simulink model "SS_Extended_Est"  (R2021a)
settings: Solver=ode45  StartTime=0.0  StopTime=1  RelTol=1e-3
undefined symbols (not defined in the file): drv, est_par, gbox, mot, rads2rpm, sens, ss_est
settings Model: Creator=gioel  LastModifiedBy=gioel
settings DataIOCC: ReturnWorkspaceOutputs=off

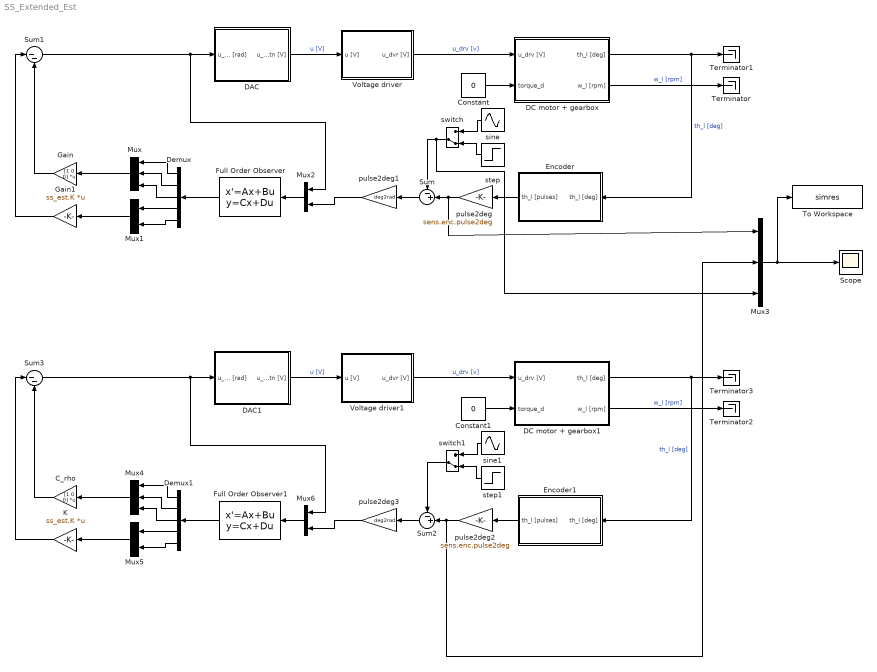
== system SS_Extended_Est ==
  C_rho : Gain  Gain=[1 0 0]  Multiplication=Matrix(K*u)
  Constant : Constant  Value=0
  Constant1 : Constant  Value=0
  DAC : Subsystem
  DAC1 : Subsystem
  DC motor + gearbox : Subsystem
  DC motor + gearbox1 : Subsystem
  Demux : Demux  Outputs=5
  Demux1 : Demux  Outputs=5
  Encoder : Subsystem
  Encoder1 : Subsystem
  Full Order Observer : StateSpace  A=ss_est.Ae_3 - ss_est.Le_3*ss_est.Ce  B=[ss_est.Be ss_est.Le_3]  C=eye(5)  D=[0 0; 0 0;0 0;0 0;0 0]  InitialCondition=0
  Full Order Observer1 : StateSpace  A=ss_est.Ae_3 - ss_est.Le_3*ss_est.Ce  B=[ss_est.Be ss_est.Le_3]  C=eye(5)  D=[0 0; 0 0;0 0;0 0;0 0]  InitialCondition=0
  Gain : Gain  Gain=[1 0 0]  Multiplication=Matrix(K*u)
  Gain1 : Gain  Gain=ss_est.K  Multiplication=Matrix(K*u)
  K : Gain  Gain=ss_est.K  Multiplication=Matrix(K*u)
  Mux : Mux  Inputs=3
  Mux{1..2,5..6} (4 alike) : Mux  Inputs=2
  Mux3 : Mux  Inputs=3
  Mux4 : Mux  Inputs=3
  Scope : Scope
  Sum : Sum  Inputs=-+|
  Sum1 : Sum  Inputs=|--
  Sum2 : Sum  Inputs=-+|
  Sum3 : Sum  Inputs=|--
  Terminator{,1..3} (4 alike) : Terminator
  To Workspace : ToWorkspace  VariableName=simres  SaveFormat=Structure With Time  SampleTime=-1
  Voltage driver : Subsystem
  Voltage driver1 : Subsystem
  pulse2deg : Gain  Gain=sens.enc.pulse2deg
  pulse2deg1 : Gain  Gain=deg2rad
  pulse2deg2 : Gain  Gain=sens.enc.pulse2deg
  pulse2deg3 : Gain  Gain=deg2rad
  sine : Sin  Amplitude=40  Frequency=2*pi/0.1  SampleTime=0
  sine1 : Sin  Amplitude=40  Frequency=2*pi/0.1  SampleTime=0
  step : Step  Time=0  After=40  SampleTime=0
  step1 : Step  Time=0  After=40  SampleTime=0
  switch : ManualSwitch  CurrentSetting=0
  switch1 : ManualSwitch  CurrentSetting=0
  wires:
  DC motor + gearbox/2(w_l [rpm]) -> Terminator/1  "w_l [rpm]"
  Voltage driver/1(u_dvr [V]) -> DC motor + gearbox/1(u_drv [V])  "u_drv [v]"
  Constant/1 -> DC motor + gearbox/2(torque_d)
  Encoder/1(th_l [pulses]) -> pulse2deg/1
  DAC/1(u_cntn [V]) -> Voltage driver/1(u [V])  "u [V]"
  Sum1/1 -> Mux2/1, DAC/1(u_dscr [rad])
  DC motor + gearbox/1(th_l [deg]) -> Terminator1/1, Encoder/1(th_l [deg])  "th_l [deg]"
  pulse2deg/1 -> Mux3/1, Sum/2
  Full Order Observer/1 -> Demux/1
  Demux/2 -> Mux/2
  Demux/1 -> Mux/1
  Demux/3 -> Mux/3
  Demux/4 -> Mux1/1
  Demux/5 -> Mux1/2
  Gain/1 -> Sum1/2
  Mux/1 -> Gain/1
  Sum/1 -> pulse2deg1/1
  pulse2deg1/1 -> Mux2/2
  Mux1/1 -> Gain1/1
  Gain1/1 -> Sum1/1
  Mux2/1 -> Full Order Observer/1
  sine/1 -> switch/1
  step/1 -> switch/2
  switch/1 -> Mux3/3, Sum/1
  switch1/1 -> Sum2/1
  step1/1 -> switch1/2
  sine1/1 -> switch1/1
  Mux6/1 -> Full Order Observer1/1
  K/1 -> Sum3/1
  Mux5/1 -> K/1
  pulse2deg3/1 -> Mux6/2
  Sum2/1 -> pulse2deg3/1
  Mux4/1 -> C_rho/1
  C_rho/1 -> Sum3/2
  Demux1/5 -> Mux5/2
  Demux1/4 -> Mux5/1
  Demux1/3 -> Mux4/3
  Demux1/1 -> Mux4/1
  Demux1/2 -> Mux4/2
  Full Order Observer1/1 -> Demux1/1
  pulse2deg2/1 -> Sum2/2, Mux3/2
  DC motor + gearbox1/1(th_l [deg]) -> Encoder1/1(th_l [deg]), Terminator3/1  "th_l [deg]"
  Sum3/1 -> DAC1/1(u_dscr [rad]), Mux6/1
  DAC1/1(u_cntn [V]) -> Voltage driver1/1(u [V])  "u [V]"
  Encoder1/1(th_l [pulses]) -> pulse2deg2/1
  Constant1/1 -> DC motor + gearbox1/2(torque_d)
  Voltage driver1/1(u_dvr [V]) -> DC motor + gearbox1/1(u_drv [V])  "u_drv [v]"
  DC motor + gearbox1/2(w_l [rpm]) -> Terminator2/1  "w_l [rpm]"
  Mux3/1 -> Scope/1, To Workspace/1

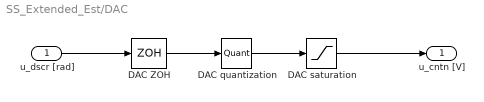
== system SS_Extended_Est/DAC ==
  u_dscr [rad] : Inport
  DAC ZOH : ZeroOrderHold  SampleTime=sens.enc.T_s
  DAC quantization : Quantizer  QuantizationInterval=daq.dac.q
  DAC saturation : Saturate  UpperLimit=10  LowerLimit=-10
  u_cntn [V] : Outport
  wires:
  DAC quantization/1 -> DAC saturation/1
  DAC ZOH/1 -> DAC quantization/1
  DAC saturation/1 -> u_cntn [V]/1
  u_dscr [rad]/1 -> DAC ZOH/1

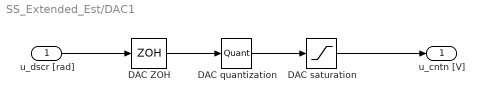
== system SS_Extended_Est/DAC1 ==
  u_dscr [rad] : Inport
  DAC ZOH : ZeroOrderHold  SampleTime=sens.enc.T_s
  DAC quantization : Quantizer  QuantizationInterval=daq.dac.q
  DAC saturation : Saturate  UpperLimit=10  LowerLimit=-10
  u_cntn [V] : Outport
  wires:
  u_dscr [rad]/1 -> DAC ZOH/1
  DAC saturation/1 -> u_cntn [V]/1
  DAC ZOH/1 -> DAC quantization/1
  DAC quantization/1 -> DAC saturation/1

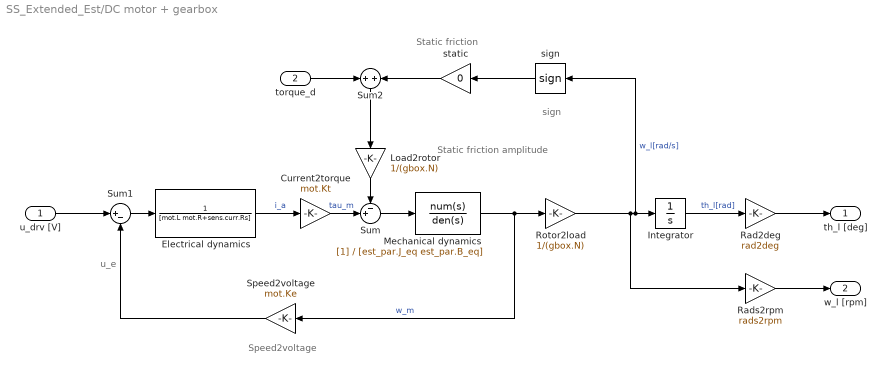
== system SS_Extended_Est/DC motor + gearbox ==
  note: u_e
  note: Speed2voltage
  note: Static friction
  note: sign
  note: Static friction
      |  amplitude
  u_drv [V] : Inport
  torque_d : Inport  Port=2
  Current2torque : Gain  Gain=mot.Kt
  Electrical dynamics : TransferFcn  Denominator=[mot.L mot.R+sens.curr.Rs]
  Integrator : Integrator
  Load2rotor : Gain  Gain=1/(gbox.N)
  Mechanical dynamics : TransferFcn  Denominator=[est_par.J_eq est_par.B_eq]
  Rad2deg : Gain  Gain=rad2deg
  Rads2rpm : Gain  Gain=rads2rpm
  Rotor2load : Gain  Gain=1/(gbox.N)
  Speed2voltage : Gain  Gain=mot.Ke
  Sum : Sum  Inputs=-+|
  Sum1 : Sum  Inputs=|+-
  Sum2 : Sum  Inputs=+|+
  sign : Signum  ZeroCross=off
  static : Gain  Gain=0
  th_l [deg] : Outport
  w_l [rpm] : Outport  Port=2
  wires:
  u_drv [V]/1 -> Sum1/1
  Rads2rpm/1 -> w_l [rpm]/1
  Electrical dynamics/1 -> Current2torque/1  "i_a"
  Current2torque/1 -> Sum/2  "tau_m"
  Rad2deg/1 -> th_l [deg]/1
  sign/1 -> static/1
  Sum1/1 -> Electrical dynamics/1
  Integrator/1 -> Rad2deg/1  "th_l[rad]"
  Sum/1 -> Mechanical dynamics/1
  Load2rotor/1 -> Sum/1
  Speed2voltage/1 -> Sum1/2
  Rotor2load/1 -> sign/1, Integrator/1, Rads2rpm/1  "w_l[rad/s]"
  Mechanical dynamics/1 -> Speed2voltage/1, Rotor2load/1  "w_m"
  Sum2/1 -> Load2rotor/1
  torque_d/1 -> Sum2/1
  static/1 -> Sum2/2

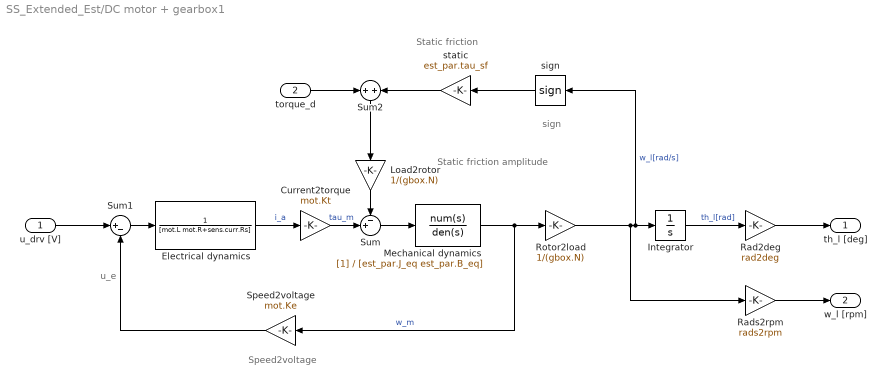
== system SS_Extended_Est/DC motor + gearbox1 ==
  note: Static friction
      |  amplitude
  note: sign
  note: Static friction
  note: Speed2voltage
  note: u_e
  u_drv [V] : Inport
  torque_d : Inport  Port=2
  Current2torque : Gain  Gain=mot.Kt
  Electrical dynamics : TransferFcn  Denominator=[mot.L mot.R+sens.curr.Rs]
  Integrator : Integrator
  Load2rotor : Gain  Gain=1/(gbox.N)
  Mechanical dynamics : TransferFcn  Denominator=[est_par.J_eq est_par.B_eq]
  Rad2deg : Gain  Gain=rad2deg
  Rads2rpm : Gain  Gain=rads2rpm
  Rotor2load : Gain  Gain=1/(gbox.N)
  Speed2voltage : Gain  Gain=mot.Ke
  Sum : Sum  Inputs=-+|
  Sum1 : Sum  Inputs=|+-
  Sum2 : Sum  Inputs=+|+
  sign : Signum  ZeroCross=off
  static : Gain  Gain=est_par.tau_sf
  th_l [deg] : Outport
  w_l [rpm] : Outport  Port=2
  wires:
  static/1 -> Sum2/2
  torque_d/1 -> Sum2/1
  Sum2/1 -> Load2rotor/1
  Mechanical dynamics/1 -> Rotor2load/1, Speed2voltage/1  "w_m"
  Rotor2load/1 -> Rads2rpm/1, Integrator/1, sign/1  "w_l[rad/s]"
  Speed2voltage/1 -> Sum1/2
  Load2rotor/1 -> Sum/1
  Sum/1 -> Mechanical dynamics/1
  Integrator/1 -> Rad2deg/1  "th_l[rad]"
  Sum1/1 -> Electrical dynamics/1
  sign/1 -> static/1
  Rad2deg/1 -> th_l [deg]/1
  Current2torque/1 -> Sum/2  "tau_m"
  Electrical dynamics/1 -> Current2torque/1  "i_a"
  Rads2rpm/1 -> w_l [rpm]/1
  u_drv [V]/1 -> Sum1/1

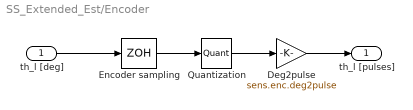
== system SS_Extended_Est/Encoder ==
  th_l [deg] : Inport
  Deg2pulse : Gain  Gain=sens.enc.deg2pulse
  Encoder sampling : ZeroOrderHold  SampleTime=0.001
  Quantization : Quantizer  QuantizationInterval=sens.enc.q
  th_l [pulses] : Outport
  wires:
  Encoder sampling/1 -> Quantization/1
  Quantization/1 -> Deg2pulse/1
  th_l [deg]/1 -> Encoder sampling/1
  Deg2pulse/1 -> th_l [pulses]/1

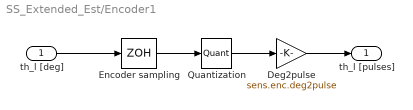
== system SS_Extended_Est/Encoder1 ==
  th_l [deg] : Inport
  Deg2pulse : Gain  Gain=sens.enc.deg2pulse
  Encoder sampling : ZeroOrderHold  SampleTime=0.001
  Quantization : Quantizer  QuantizationInterval=sens.enc.q
  th_l [pulses] : Outport
  wires:
  Deg2pulse/1 -> th_l [pulses]/1
  th_l [deg]/1 -> Encoder sampling/1
  Quantization/1 -> Deg2pulse/1
  Encoder sampling/1 -> Quantization/1

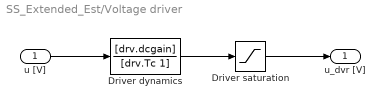
== system SS_Extended_Est/Voltage driver ==
  u [V] : Inport
  Driver dynamics : TransferFcn  Numerator=[drv.dcgain]  Denominator=[drv.Tc 1]
  Driver saturation : Saturate  UpperLimit=12  LowerLimit=-12
  u_dvr [V] : Outport
  wires:
  Driver saturation/1 -> u_dvr [V]/1
  Driver dynamics/1 -> Driver saturation/1
  u [V]/1 -> Driver dynamics/1

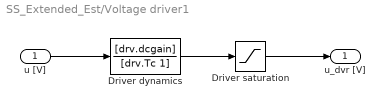
== system SS_Extended_Est/Voltage driver1 ==
  u [V] : Inport
  Driver dynamics : TransferFcn  Numerator=[drv.dcgain]  Denominator=[drv.Tc 1]
  Driver saturation : Saturate  UpperLimit=12  LowerLimit=-12
  u_dvr [V] : Outport
  wires:
  u [V]/1 -> Driver dynamics/1
  Driver dynamics/1 -> Driver saturation/1
  Driver saturation/1 -> u_dvr [V]/1
